simulink model "SST_MMC"  (R2014a)
settings: Solver=ode45  StartTime=0.0  StopTime=0.2  RelTol=1e-3
libraries: powerlib x328, simulink x1
(part 3 of 3)

== system SST_MMC/MMC_6_SM/arm6/sm6 ==
  " GATE_SIGNAL " : Inport
  " " : powerlib/Measurements/Current Measurement  PhasorSimulation=off  OutputType=Complex  PSBequivalent=0
  " 1" : powerlib/Measurements/Current Measurement  PhasorSimulation=off  OutputType=Complex  PSBequivalent=0
  " 2" : powerlib/Measurements/Current Measurement  PhasorSimulation=off  OutputType=Complex  PSBequivalent=0
  C_SM : powerlib/Elements/Series RLC Branch  LConnTagsString=__new0  RConnTagsString=__new0  BranchType=C  Resistance=1  Inductance=1e-3  SetiL0=off  InitialCurrent=0  Capacitance=C_SM  Setx0=on  InitialVoltage=VC_SM  Measurements=None
  Logical Operator : Logic  Operator=NOT  AllPortsSameDT=off  OutDataTypeStr=boolean
  Mux : Mux  Inputs=2
  Mux1 : Mux  Inputs=2
  VC : powerlib/Measurements/Voltage Measurement  PhasorSimulation=off  OutputType=Complex  PSBequivalent=0
  VC1 : powerlib/Measurements/Voltage Measurement  PhasorSimulation=off  OutputType=Complex  PSBequivalent=0
  VC_GRAPH : Scope
  sw1 : powerlib/Power Electronics/IGBT//Diode  Ron=Ron  Rs=1e5  Cs=inf  Measurements=off
  sw2 : powerlib/Power Electronics/IGBT//Diode  Ron=Ron  Rs=1e5  Cs=inf  Measurements=off
  POSITIVE : PMIOPort  Port=1  Side=Right
  NEGATIVE : PMIOPort  Port=2  Side=Right
  " VC_S_M" : Outport
  " c_ce" : Outport  Port=2
  " smvi" : Outport  Port=3
  wires:
  VC/1 -> " VC_S_M"/1, VC_GRAPH/1
  Logical Operator/1 -> sw1/1
  " GATE_SIGNAL "/1 -> Logical Operator/1, sw2/1
  " 1"/1 -> Mux1/1
  " 2"/1 -> Mux1/2
  " "/1 -> Mux/1
  VC1/1 -> Mux/2
  Mux1/1 -> " c_ce"/1
  Mux/1 -> " smvi"/1
  connections:
  sw1/RConn1 -- " 2"/LConn1
  VC/LConn2 -- C_SM/RConn1 -- sw2/RConn1 -- NEGATIVE/RConn1 -- VC1/LConn2
  VC/LConn1 -- C_SM/LConn1 -- " 1"/RConn1
  POSITIVE/RConn1 -- " "/LConn1 -- VC1/LConn1
  " 1"/LConn1 -- sw1/LConn1
  " 2"/RConn1 -- sw2/LConn1 -- " "/RConn1

== matlab function SST_MMC/CONTROL BLOCK/DAB CONTROL ==
  data: sig_ref output; t input
function sig_ref  = fcn(t)

%% parameters for DAB SST
Tsw=2*5e-5;%%switching perod;
NRs=rem(round(t/Tsw),2);

%% reference signal creation
if(NRs==0)
    sig_ref=1;
else
    sig_ref=0;
end

== matlab function SST_MMC/CONTROL BLOCK/MMC CONTROL ==
  data: ia input; sa output size=[1 12]; ib input; ic input; va input; vb input; vc input; sb output size=[1 12]; sc output size=[1 12]
function [sa,sb,sc]=fcn(ia,ib,ic,va,vb,vc)
%% parameters
n=6;%% number of submodules
s=ones(1,n);
Vcap=3e3;
Ts=5e-5;
Csm=10e-3;
dV=100;%%allowed ripple in cpacitance

l=load('m');
%% coefficients of eular approximation equations
Kv=Ts/Csm;%%Vu(t+Ts)=Vu(t)+Kv*iu(t)

%% capacitor voltages
vua=va(1:n)';
vla=va(n+1:2*n)';
vub=vb(1:n)';
vlb=vb(n+1:2*n)';
vuc=vc(1:n)';
vlc=vc(n+1:2*n)';
%% arm currents
iua=ia(1);
ila=ia(2);
iub=ib(1);
ilb=ib(2);
iuc=ic(1);
ilc=ic(2);
%% voltage balancing and sorting
%%   phase a
  i=iua;
  vu=vua;
  vl=vla;
  v1a=s;
  v2a=s;
  iu=iua;
  il=ila;
  VC=max([vu-Vcap vl-Vcap]);
if(VC>dV)
  [~,ui]=sort(vu-Vcap);
  [~,li]=sort(vl-Vcap);
  if(i>=0)
    v1a(ui(1:n/2))=0;
    v2a(li(n/2+1:n))=0;
  else
    v1a(ui(n/2+1:n))=0;
    v2a(li(1:n/2))=0;
  end
  vsa=[v1a v2a];
else
    e=zeros(1,length(l.sm));
    for ii=1:length(l.sm)
      vun=vu+Kv*iu*l.sm(ii,1:n);
      vln=vl+Kv*il*l.sm(ii,n+1:2*n);
      Vdcn=sum(vun)+sum(vln);
      e(ii)=abs(n*Vcap-Vdcn);
    end
    [~,o]=min(e);
    vsa=l.sm(o,:);
end
%%   phase b
  i=iub;
  vu=vub;
  vl=vlb;
  v1b=s;
  v2b=s;
  iu=iub;
  il=ilb;
  VC=max([vu-Vcap vl-Vcap]);
if(VC>dV)
  [~,ui]=sort(vu-Vcap);
  [~,li]=sort(vl-Vcap);
  if(i>=0)
    v1b(ui(1:n/2))=0;
    v2b(li(n/2+1:n))=0;
  else
    v1b(ui(n/2+1:n))=0;
    v2b(li(1:n/2))=0;
  end
  vsb=[v1b v2b];
else
    e=zeros(1,length(l.sm));
    for ii=1:length(l.sm)
      vun=vu+Kv*iu*l.sm(ii,1:n);
      vln=vl+Kv*il*l.sm(ii,n+1:2*n);
      Vdcn=sum(vun)+sum(vln);
      e(ii)=abs(n*Vcap-Vdcn);
    end
    [~,o]=min(e);
    vsb=l.sm(o,:);
end

%%   phase c
  i=iuc;
  vu=vuc;
  vl=vlc;
  v1c=s;
  v2c=s;
  iu=iuc;
  il=ilc;
  VC=max([vu-Vcap vl-Vcap]);
if(VC>dV)
  [~,ui]=sort(vu-Vcap);
  [~,li]=sort(vl-Vcap);
  if(i>=0)
    v1c(ui(1:n/2))=0;
    v2c(li(n/2+1:n))=0;
  else
    v1c(ui(n/2+1:n))=0;
    v2c(li(1:n/2))=0;
  end
  vsc=[v1c v2c];
else
    e=zeros(1,length(l.sm));
    for ii=1:length(l.sm)
      vun=vu+Kv*iu*l.sm(ii,1:n);
      vln=vl+Kv*il*l.sm(ii,n+1:2*n);
      Vdcn=sum(vun)+sum(vln);
      e(ii)=abs(n*Vcap-Vdcn);
    end
    [~,o]=min(e);
    vsc=l.sm(o,:);
end

%%  
sa=vsa(1:end);
sb=vsb(1:end);
sc=vsc(1:end);

== matlab function SST_MMC/CONTROL BLOCK/Inverter Control ==
  data: t input; Pa output; Pb output; Pc output; RL input; LL input
function [Pa,Pb,Pc]= fcn(t,RL,LL)
%% reference carrier
w=2*pi*60;
Zeq=complex(RL,w*LL);
O=angle(Zeq);
Pa=sin(w*t);
Pb=sin(w*t+2*pi/3);
Pc=sin(w*t-2*pi/3);
